simulink model "bmex"  (Simulink 8.5)
settings: Solver=ode45  SolverMode=SingleTasking  StartTime=0.0  StopTime=0.25  FixedStep=1/1200  RelTol=1e-3  AbsTol=1e-6
libraries: elements x6, inputs x2
settings Model: Creator=PC  LastModifiedBy=PC
settings DataIOCC: LimitDataPoints=off
settings OptimizationCC: BlockReduction=off  BooleanDataType=off  ExpressionDepthLimit=128
settings DebuggingCC: SaveWithParameterizedLinksMsg=none  SignalResolutionControl=TryResolveAllWithWarning  MultiTaskDSMMsg=warning  MultiTaskCondExecSysMsg=none  FcnCallInpInsideContextMsg=EnableAllAsError  StateNameClashWarn=none
settings HardwareCC: TargetUnknown=on
settings RTWCC: TemplateMakefile=grt_unix.tmf

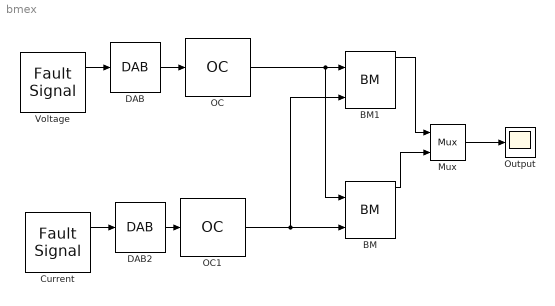
== system bmex ==
  BM : elements/BM  tpostv=median  plenv=40  tposti=median  pleni=10  tposts=mean  plens=20  tpostz=none  plenz=10
  BM1 : elements/BM  tpostv=none  plenv=5  tposti=median  pleni=10  tposts=mean  plens=20  tpostz=median  plenz=10
  Current : inputs/Fault Signal  pre_fault=[4 45]  post_fault=[10 90]  fr_dc=[60 1.25/60 0.0004]  oscA=[2.0 0.8 0.9]  oscf=[800 1000 3000]  oscT=[0.050 0.30 0.060]
  DAB : elements/DAB  filter=on  approx=Bessel  order=2  numerator=[]  denominator=[]  freq=200  resdis=off  vertres=12  xmax=10  winsize=40  G=1.0  fs=60*40
  DAB2 : elements/DAB  filter=on  approx=Bessel  order=2  numerator=[]  denominator=[]  freq=200  resdis=off  vertres=12  xmax=10  winsize=40  G=1.0  fs=60*40
  Mux : Mux  Inputs=2
  OC : elements/OC  tfilt=Fourier  rfilt=[ ]  ifilt=[ ]  tlen=full  N1=40
  OC1 : elements/OC  tfilt=Fourier  rfilt=[ ]  ifilt=[ ]  tlen=full  N1=40
  "Output " : Scope
      settings: TickLabels=on  YMin=2  YMax=7.5
  Voltage : inputs/Fault Signal  pre_fault=[7 45]  post_fault=[4 90]  fr_dc=[60 5/60 0.05]  oscA=[1 1.0 0.8 0.9]  oscf=[ 0 800 1000 3000]  oscT=[ 0.004 0.50 0.030 0.060]
  wires:
  DAB/1 -> OC/1
  DAB2/1 -> OC1/1
  OC1/1 -> BM/2, BM1/2
  Mux/1 -> "Output "/1
  BM/1 -> Mux/2
  Current/1 -> DAB2/1
  Voltage/1 -> DAB/1
  OC/1 -> BM/1, BM1/1
  BM1/1 -> Mux/1
